simulink model "Flight_Simulation"  (R2021b)
settings: Solver=ode4  StartTime=0.0  StopTime=20  FixedStep=Settings.Simulation.step_size  RelTol=1e-3  EnableMultiTasking=on
undefined symbols (not defined in the file or in its folder): AeroCoeff, Aircraft, ControlGains, dLEF, Environment, F, Light, MIL, Settings, Trim, trim_control, trim_state, trim_thrust
libraries: simulink x19, simulink_extras x14, slpidlib x2, aerolibfltsims x2, aerolibwind2 x1, vrlib x1
(part 4 of 5)

== system Flight_Simulation/Non-linear_Plant/6DOF_Equations/Position_Differential_Equations/Calculate_north_position_dot ==
  U : Inport
  V : Inport  Port=2
  W : Inport  Port=3
  phi : Inport  Port=4
  theta : Inport  Port=5
  psi : Inport  Port=6
  Product3 : Product  Inputs=3
  Product4 : Product  Inputs=3
  Product{5..6,8..9} (4 alike) : Product
  Product7 : Product  Inputs=3
  Sum : Sum  Inputs=+-
  Sum1 : Sum
  Sum2 : Sum  Inputs=+++
  Trigonometric Function4 : Trigonometry  Operator=cos
  Trigonometric Function5 : Trigonometry  Operator=cos
  Trigonometric Function6 : Trigonometry
  Trigonometric Function7 : Trigonometry
  Trigonometric Function8 : Trigonometry  Operator=cos
  Trigonometric Function9 : Trigonometry
  north_pos_dot : Outport
  wires:
  phi/1 -> Trigonometric Function6/1, Trigonometric Function5/1
  Trigonometric Function7/1 -> Product7/2, Product4/3
  Product5/1 -> Sum/2
  V/1 -> Product6/1
  U/1 -> Product3/1
  W/1 -> Product9/1
  Trigonometric Function6/1 -> Product8/1, Product4/1
  psi/1 -> Trigonometric Function9/1, Trigonometric Function8/1
  Product3/1 -> Sum2/1
  Sum/1 -> Product6/2
  Trigonometric Function9/1 -> Product8/2, Product5/2
  Trigonometric Function8/1 -> Product4/2, Product3/3, Product7/3
  Trigonometric Function5/1 -> Product7/1, Product5/1
  Product7/1 -> Sum1/1
  Trigonometric Function4/1 -> Product3/2
  theta/1 -> Trigonometric Function7/1, Trigonometric Function4/1
  Sum1/1 -> Product9/2
  Product4/1 -> Sum/1
  Product9/1 -> Sum2/3
  Sum2/1 -> north_pos_dot/1  "north_pos_dot_m/s"
  Product6/1 -> Sum2/2
  Product8/1 -> Sum1/2

== system Flight_Simulation/Non-linear_Plant/6DOF_Equations/Position_Differential_Equations/Position_dot_WGS84 ==
  U_earth : Inport
  V_earth : Inport  Port=2
  alt_dot : Inport  Port=3
  Pos_WGS84 : Inport  Port=4
  Earth_Model_BUS : Inport  Port=5
  Bus Creator : BusCreator  Inputs=3
  Bus Selector : BusSelector  OutputSignals=R_Curvature_Meridian_m,R_Curvature_Prime_Vertical_m
  Bus Selector1 : BusSelector  OutputSignals=mue_pos_WGS84_rad,h_pos_WGS84_m
  Gain : Gain
  Product : Product
  Product1 : Product  Inputs=*/
  Product2 : Product  Inputs=*/
  Sum : Sum  Inputs=|++
  Sum1 : Sum
  Trigonometric Function : Trigonometry  Operator=cos
  Pos_WGS84_dot_BUS : Outport
  wires:
  Trigonometric Function/1 -> Product/1
  Sum/1 -> Product/2
  Bus Selector1/2 -> Sum1/1, Sum/1  "<h_pos_WGS84_m>"
  Bus Selector1/1 -> Trigonometric Function/1  "<mue_pos_WGS84_rad>"
  Product/1 -> Product1/2
  Earth_Model_BUS/1 -> Bus Selector/1
  Bus Selector/1 -> Sum1/2  "<R_Curvature_Meridian_m>"
  Bus Selector/2 -> Sum/2  "<R_Curvature_Prime_Vertical_m>"
  Sum1/1 -> Product2/2
  Product1/1 -> Bus Creator/1  "Pos_lambda_dot_WGS84_rad/s"
  Product2/1 -> Bus Creator/2  "Pos_mue_dot_WGS84_rad/s"
  Gain/1 -> Bus Creator/3  "Pos_h_dot_WGS84_m/s"
  Bus Creator/1 -> Pos_WGS84_dot_BUS/1  "Pos_WGS84_dot_BUS"
  V_earth/1 -> Product1/1
  U_earth/1 -> Product2/1
  alt_dot/1 -> Gain/1
  Pos_WGS84/1 -> Bus Selector1/1

== system Flight_Simulation/Non-linear_Plant/6DOF_Equations/Rotation_Differential_Equation/Inertia_Denominator_Calculation ==
  Aircraft_Constants_BUS : Inport
  Add : Sum  Inputs=+-
  Bus Selector : BusSelector  OutputSignals=Mass_Properties_BUS
  Bus Selector1 : BusSelector  OutputSignals=J_xx_kg*m^2,J_zz_kg*m^2,J_xz_kg*m^2
  Product : Product
  Product1 : Product
  Inertia_Denominator : Outport
  wires:
  Aircraft_Constants_BUS/1 -> Bus Selector/1
  Bus Selector/1 -> Bus Selector1/1  "<Mass_Properties_BUS>"
  Bus Selector1/1 -> Product/1  "<J_xx_kg*m^2>"
  Bus Selector1/2 -> Product/2  "<J_zz_kg*m^2>"
  Product/1 -> Add/1
  Bus Selector1/3 -> Product1/2, Product1/1  "<J_xz_kg*m^2>"
  Product1/1 -> Add/2
  Add/1 -> Inertia_Denominator/1

== system Flight_Simulation/Non-linear_Plant/6DOF_Equations/Rotation_Differential_Equation/p_dot_Calculation ==
  Moments_total_BUS : Inport
  Aircraft_Constants_BUS : Inport  Port=2
  States_BUS : Inport  Port=3
  Inertia_Denominator : Inport  Port=4
  Add : Sum  Inputs=++-++
  Add1 : Sum  Inputs=-+
  Add2 : Sum
  Add3 : Sum  Inputs=+-+
  Bus Selector : BusSelector  OutputSignals=Rates_p_q_r
  Bus Selector1 : BusSelector  OutputSignals=p_rad/s,q_rad/s,r_rad/s
  Bus Selector2 : BusSelector  OutputSignals=Engine_Const_BUS,Mass_Properties_BUS
  Bus Selector3 : BusSelector  OutputSignals=J_xx_kg*m^2,J_yy_kg*m^2,J_zz_kg*m^2,J_xz_kg*m^2
  Bus Selector4 : BusSelector  OutputSignals=L_total,N_total
  Bus Selector5 : BusSelector  OutputSignals=Engine_Ang_Mom_kg*m^2/s
  Divide : Product  Inputs=*/
  Product{,1..3} (4 alike) : Product
  Product4 : Product  Inputs=3
  Product5 : Product  Inputs=4
  Product6 : Product  Inputs=3
  p_dot : Outport
  wires:
  States_BUS/1 -> Bus Selector/1
  Bus Selector/1 -> Bus Selector1/1  "<Rates_p_q_r>"
  Aircraft_Constants_BUS/1 -> Bus Selector2/1
  Bus Selector2/2 -> Bus Selector3/1  "<Mass_Properties_BUS>"
  Moments_total_BUS/1 -> Bus Selector4/1
  Bus Selector3/4 -> Product6/3, Product5/2, Product3/1, Product3/2, Product1/1  "<J_xz_kg*m^2>"
  Bus Selector3/3 -> Add3/3, Product2/2, Add1/2, Product/1  "<J_zz_kg*m^2>"
  Bus Selector4/1 -> Product/2  "<L_total>"
  Bus Selector4/2 -> Product1/2  "<N_total>"
  Product/1 -> Add/4  "Jzz_L"
  Product1/1 -> Add/5  "Jxz_N"
  Add/1 -> Divide/1
  Bus Selector3/2 -> Add3/2, Add1/1  "<J_yy_kg*m^2>"
  Add1/1 -> Product2/1
  Product2/1 -> Add2/2
  Product3/1 -> Add2/1
  Add2/1 -> Product4/3
  Bus Selector1/2 -> Product6/2, Product5/4, Product4/1  "<q_rad/s>"
  Bus Selector1/3 -> Product4/2  "<r_rad/s>"
  Product4/1 -> Add/3  "QR_term"
  Bus Selector3/1 -> Add3/1  "<J_xx_kg*m^2>"
  Add3/1 -> Product5/1
  Bus Selector1/1 -> Product5/3  "<p_rad/s>"
  Product5/1 -> Add/2  "PQ_term"
  Product6/1 -> Add/1
  Bus Selector2/1 -> Bus Selector5/1  "<Engine_Const_BUS>"
  Bus Selector5/1 -> Product6/1  "<Engine_Ang_Mom_kg*m^2/s>"
  Inertia_Denominator/1 -> Divide/2
  Divide/1 -> p_dot/1  "p_dot_rad/s^2"

== system Flight_Simulation/Non-linear_Plant/6DOF_Equations/Rotation_Differential_Equation/q_dot_Calculation ==
  note: * Momentum_engine_angular
  States_BUS : Inport
  Aircraft_Constants_BUS : Inport  Port=2
  Moments_total_BUS : Inport  Port=3
  Engine_BUS : Inport  Port=4
  Add : Sum  Inputs=-+-+
  Add1 : Sum  Inputs=-+
  Add2 : Sum  Inputs=+-
  Bus Selector : BusSelector  OutputSignals=Rates_p_q_r
  Bus Selector1 : BusSelector  OutputSignals=p_rad/s,r_rad/s
  Bus Selector2 : BusSelector  OutputSignals=Engine_Const_BUS,Mass_Properties_BUS
  Bus Selector3 : BusSelector  OutputSignals=J_xx_kg*m^2,J_zz_kg*m^2,J_xz_kg*m^2,J_yy_kg*m^2
  Bus Selector4 : BusSelector  OutputSignals=M_total
  Bus Selector5 : BusSelector  OutputSignals=Engine_Ang_Mom_kg*m^2/s
  Bus Selector6 : BusSelector  OutputSignals=M_engine_Nm
  Divide : Product  Inputs=*/
  Product : Product  Inputs=3
  Product{1..4} (4 alike) : Product
  Sum : Sum  Inputs=|++
  q_dot : Outport
  wires:
  Divide/1 -> q_dot/1  "q_dot_rad/s^2"
  Bus Selector2/1 -> Bus Selector5/1  "<Engine_Const_BUS>"
  Add/1 -> Divide/1
  Moments_total_BUS/1 -> Bus Selector4/1
  Bus Selector2/2 -> Bus Selector3/1  "<Mass_Properties_BUS>"
  Aircraft_Constants_BUS/1 -> Bus Selector2/1
  Bus Selector/1 -> Bus Selector1/1  "<Rates_p_q_r>"
  States_BUS/1 -> Bus Selector/1
  Bus Selector4/1 -> Sum/1  "<M_total>"
  Bus Selector3/1 -> Add1/1  "<J_xx_kg*m^2>"
  Bus Selector3/2 -> Add1/2  "<J_zz_kg*m^2>"
  Add1/1 -> Product/3
  Bus Selector1/1 -> Product2/1, Product2/2, Product/1  "<p_rad/s>"
  Bus Selector1/2 -> Product4/2, Product3/1, Product3/2, Product/2  "<r_rad/s>"
  Product/1 -> Add/2  "PR_term"
  Bus Selector3/3 -> Product1/2  "<J_xz_kg*m^2>"
  Product2/1 -> Add2/1
  Product3/1 -> Add2/2
  Add2/1 -> Product1/1
  Product1/1 -> Add/3  "jxz_term"
  Bus Selector5/1 -> Product4/1  "<Engine_Ang_Mom_kg*m^2/s>"
  Product4/1 -> Add/1
  Bus Selector3/4 -> Divide/2  "<J_yy_kg*m^2>"
  Sum/1 -> Add/4  "M_total+M_engine"
  Engine_BUS/1 -> Bus Selector6/1
  Bus Selector6/1 -> Sum/2  "<M_engine_Nm>"

== system Flight_Simulation/Non-linear_Plant/6DOF_Equations/Rotation_Differential_Equation/r_dot_Calculation ==
  Inertia_Denominator : Inport
  States_BUS : Inport  Port=2
  Aircraft_Constants_BUS : Inport  Port=3
  Moments_total_BUS : Inport  Port=4
  Add : Sum  Inputs=+-+++
  Add1 : Sum  Inputs=+-
  Add2 : Sum
  Add3 : Sum  Inputs=+-+
  Bus Selector : BusSelector  OutputSignals=Rates_p_q_r
  Bus Selector1 : BusSelector  OutputSignals=p_rad/s,q_rad/s,r_rad/s
  Bus Selector2 : BusSelector  OutputSignals=Engine_Const_BUS,Mass_Properties_BUS
  Bus Selector3 : BusSelector  OutputSignals=J_xx_kg*m^2,J_yy_kg*m^2,J_zz_kg*m^2,J_xz_kg*m^2
  Bus Selector4 : BusSelector  OutputSignals=L_total,N_total
  Bus Selector5 : BusSelector  OutputSignals=Engine_Ang_Mom_kg*m^2/s
  Divide : Product  Inputs=*/
  Product{,1..3} (4 alike) : Product
  Product4 : Product  Inputs=3
  Product5 : Product  Inputs=4
  Product6 : Product  Inputs=3
  r_dot : Outport
  wires:
  Divide/1 -> r_dot/1  "r_dot_rad/s^2"
  Inertia_Denominator/1 -> Divide/2
  Bus Selector5/1 -> Product6/1  "<Engine_Ang_Mom_kg*m^2/s>"
  Bus Selector2/1 -> Bus Selector5/1  "<Engine_Const_BUS>"
  Product6/1 -> Add/1
  Product5/1 -> Add/2
  Add3/1 -> Product5/1
  Product4/1 -> Add/3  "PQ_Term"
  Add2/1 -> Product4/3
  Product3/1 -> Add2/1
  Product2/1 -> Add2/2
  Add1/1 -> Product2/1
  Add/1 -> Divide/1
  Product1/1 -> Add/5  "Jx_N"
  Product/1 -> Add/4  "Jxz_L"
  Moments_total_BUS/1 -> Bus Selector4/1
  Bus Selector2/2 -> Bus Selector3/1  "<Mass_Properties_BUS>"
  Aircraft_Constants_BUS/1 -> Bus Selector2/1
  Bus Selector/1 -> Bus Selector1/1  "<Rates_p_q_r>"
  States_BUS/1 -> Bus Selector/1
  Bus Selector4/2 -> Product1/2  "<N_total>"
  Bus Selector3/1 -> Product6/3, Add3/1, Add1/1, Product2/2, Product1/1  "<J_xx_kg*m^2>"
  Bus Selector3/4 -> Product5/4, Product3/1, Product3/2, Product/1  "<J_xz_kg*m^2>"
  Bus Selector4/1 -> Product/2  "<L_total>"
  Bus Selector3/2 -> Add3/2, Add1/2  "<J_yy_kg*m^2>"
  Bus Selector1/1 -> Product4/1  "<p_rad/s>"
  Bus Selector1/2 -> Product6/2, Product5/2, Product4/2  "<q_rad/s>"
  Bus Selector3/3 -> Add3/3  "<J_zz_kg*m^2>"
  Bus Selector1/3 -> Product5/3  "<r_rad/s>"

== system Flight_Simulation/Non-linear_Plant/6DOF_Equations/Translation_UVW_Differential_Equations/U_dot ==
  States_BUS : Inport
  Forces_total_BUS : Inport  Port=2
  Aircraft_Constants_BUS : Inport  Port=3
  Gravity_BUS : Inport  Port=4
  Engine_BUS : Inport  Port=5
  Bus Selector : BusSelector  OutputSignals=Angles_phi_theta_psi
  Bus Selector1 : BusSelector  OutputSignals=theta_rad
  Bus Selector10 : BusSelector  OutputSignals=X_total
  Bus Selector11 : BusSelector  OutputSignals=Thrust_act_N
  Bus Selector2 : BusSelector  OutputSignals=g_m/s^2
  Bus Selector3 : BusSelector  OutputSignals=Rates_p_q_r
  Bus Selector4 : BusSelector  OutputSignals=q_rad/s,r_rad/s
  Bus Selector5 : BusSelector  OutputSignals=V_m/s,W_m/s
  Bus Selector6 : BusSelector  OutputSignals=Vel_U_V_W_body
  Bus Selector9 : BusSelector  OutputSignals=Mass_Properties_BUS.Mass_kg
  Divide : Product  Inputs=/*
  Divide1 : Product  Inputs=*/
  Product : Product
  Product1 : Product
  Product2 : Product
  Sum : Sum  Inputs=--+++
  Trigonometric Function : Trigonometry
  U_dot : Outport
  wires:
  Sum/1 -> U_dot/1  "U_dot"
  States_BUS/1 -> Bus Selector3/1, Bus Selector6/1, Bus Selector/1
  Bus Selector/1 -> Bus Selector1/1  "<Angles_phi_theta_psi>"
  Bus Selector1/1 -> Trigonometric Function/1  "<theta_rad>"
  Gravity_BUS/1 -> Bus Selector2/1
  Bus Selector2/1 -> Product/1  "<g_m/s^2>"
  Trigonometric Function/1 -> Product/2
  Product/1 -> Sum/1
  Bus Selector3/1 -> Bus Selector4/1  "<Rates_p_q_r>"
  Bus Selector4/1 -> Product2/1  "<q_rad/s>"
  Bus Selector4/2 -> Product1/1  "<r_rad/s>"
  Bus Selector5/1 -> Product1/2  "<V_m/s>"
  Product1/1 -> Sum/3
  Bus Selector5/2 -> Product2/2  "<W_m/s>"
  Product2/1 -> Sum/2
  Aircraft_Constants_BUS/1 -> Bus Selector9/1
  Bus Selector9/1 -> Divide1/2, Divide/1  "<Mass_kg>"
  Forces_total_BUS/1 -> Bus Selector10/1
  Engine_BUS/1 -> Bus Selector11/1
  Bus Selector11/1 -> Divide1/1  "<Thrust_act_N>"
  Bus Selector10/1 -> Divide/2  "<X_total>"
  Divide/1 -> Sum/5
  Divide1/1 -> Sum/4
  Bus Selector6/1 -> Bus Selector5/1  "<Vel_U_V_W_body>"

== system Flight_Simulation/Non-linear_Plant/6DOF_Equations/Translation_UVW_Differential_Equations/V_dot ==
  States_BUS : Inport
  Forces_total_BUS : Inport  Port=2
  Aircraft_Constants_BUS1 : Inport  Port=3
  Gravity_BUS : Inport  Port=4
  Bus Selector : BusSelector  OutputSignals=Angles_phi_theta_psi
  Bus Selector1 : BusSelector  OutputSignals=phi_rad,theta_rad
  Bus Selector11 : BusSelector  OutputSignals=Y_total
  Bus Selector12 : BusSelector  OutputSignals=Mass_Properties_BUS.Mass_kg
  Bus Selector2 : BusSelector  OutputSignals=g_m/s^2
  Bus Selector3 : BusSelector  OutputSignals=Rates_p_q_r
  Bus Selector4 : BusSelector  OutputSignals=p_rad/s,r_rad/s
  Bus Selector5 : BusSelector  OutputSignals=U_m/s,W_m/s
  Bus Selector6 : BusSelector  OutputSignals=Vel_U_V_W_body
  Divide1 : Product  Inputs=/*
  Product : Product  Inputs=3
  Product1 : Product
  Product2 : Product
  Sum : Sum  Inputs=++-+
  Trigonometric Function : Trigonometry
  Trigonometric Function1 : Trigonometry  Operator=cos
  V_dot : Outport
  wires:
  Sum/1 -> V_dot/1  "V_dot"
  States_BUS/1 -> Bus Selector6/1, Bus Selector3/1, Bus Selector/1
  Bus Selector/1 -> Bus Selector1/1  "<Angles_phi_theta_psi>"
  Bus Selector1/2 -> Trigonometric Function1/1  "<theta_rad>"
  Gravity_BUS/1 -> Bus Selector2/1
  Bus Selector2/1 -> Product/1  "<g_m/s^2>"
  Trigonometric Function/1 -> Product/2
  Product/1 -> Sum/1  "g_ct_sphi"
  Bus Selector3/1 -> Bus Selector4/1  "<Rates_p_q_r>"
  Bus Selector4/1 -> Product2/1  "<p_rad/s>"
  Bus Selector4/2 -> Product1/1  "<r_rad/s>"
  Bus Selector5/1 -> Product1/2  "<U_m/s>"
  Product1/1 -> Sum/3  "RU"
  Bus Selector5/2 -> Product2/2  "<W_m/s>"
  Product2/1 -> Sum/2  "PW"
  Trigonometric Function1/1 -> Product/3
  Bus Selector1/1 -> Trigonometric Function/1  "<phi_rad>"
  Divide1/1 -> Sum/4  "qbar_S_Cy_m"
  Forces_total_BUS/1 -> Bus Selector11/1
  Bus Selector12/1 -> Divide1/1  "<Mass_kg>"
  Bus Selector11/1 -> Divide1/2  "<Y_total>"
  Aircraft_Constants_BUS1/1 -> Bus Selector12/1
  Bus Selector6/1 -> Bus Selector5/1  "<Vel_U_V_W_body>"

== system Flight_Simulation/Non-linear_Plant/6DOF_Equations/Translation_UVW_Differential_Equations/W_dot ==
  States_BUS : Inport
  Force_Coeff_BUS : Inport  Port=2
  Aircraft_Constants_BUS : Inport  Port=3
  Gravity_BUS : Inport  Port=4
  Bus Selector : BusSelector  OutputSignals=Angles_phi_theta_psi
  Bus Selector1 : BusSelector  OutputSignals=phi_rad,theta_rad
  Bus Selector10 : BusSelector  OutputSignals=Z_total
  Bus Selector2 : BusSelector  OutputSignals=g_m/s^2
  Bus Selector3 : BusSelector  OutputSignals=Rates_p_q_r
  Bus Selector4 : BusSelector  OutputSignals=q_rad/s,p_rad/s
  Bus Selector5 : BusSelector  OutputSignals=V_m/s,U_m/s
  Bus Selector6 : BusSelector  OutputSignals=Vel_U_V_W_body
  Bus Selector9 : BusSelector  OutputSignals=Mass_Properties_BUS.Mass_kg
  Divide : Product  Inputs=*/
  Product : Product  Inputs=3
  Product1 : Product
  Product2 : Product
  Sum : Sum  Inputs=++-+
  Trigonometric Function : Trigonometry  Operator=cos
  Trigonometric Function1 : Trigonometry  Operator=cos
  W_dot : Outport
  wires:
  Aircraft_Constants_BUS/1 -> Bus Selector9/1
  Product2/1 -> Sum/2  "UQ"
  Bus Selector5/2 -> Product2/2  "<U_m/s>"
  Product1/1 -> Sum/3  "VP"
  Bus Selector5/1 -> Product1/2  "<V_m/s>"
  Bus Selector4/2 -> Product1/1  "<p_rad/s>"
  Bus Selector4/1 -> Product2/1  "<q_rad/s>"
  Bus Selector3/1 -> Bus Selector4/1  "<Rates_p_q_r>"
  Product/1 -> Sum/1  "g_ctheta_cphi"
  Trigonometric Function/1 -> Product/3
  Bus Selector2/1 -> Product/1  "<g_m/s^2>"
  Gravity_BUS/1 -> Bus Selector2/1
  Bus Selector1/2 -> Trigonometric Function/1  "<theta_rad>"
  Bus Selector/1 -> Bus Selector1/1  "<Angles_phi_theta_psi>"
  States_BUS/1 -> Bus Selector/1, Bus Selector6/1, Bus Selector3/1
  Sum/1 -> W_dot/1  "W_dot"
  Divide/1 -> Sum/4  "Z_total/m"
  Bus Selector1/1 -> Trigonometric Function1/1  "<phi_rad>"
  Trigonometric Function1/1 -> Product/2
  Bus Selector9/1 -> Divide/2  "<Mass_kg>"
  Bus Selector10/1 -> Divide/1  "<Z_total>"
  Force_Coeff_BUS/1 -> Bus Selector10/1
  Bus Selector6/1 -> Bus Selector5/1  "<Vel_U_V_W_body>"

== system Flight_Simulation/Non-linear_Plant/Actuator_Models/Leading Edge Flap/LEF Actuator ==
  In1 : Inport
  Command Saturation : Saturate  UpperLimit=25  LowerLimit=0
  Gain : Gain  Gain=1/0.136  SaturateOnIntegerOverflow=on  OutDataTypeStr=Inherit: Same as input  ParamDataTypeStr=Inherit: Same as input
  "LF_pos_int " : Integrator  InitialConditionSource=external  InitialCondition=dLEF  UpperSaturationLimit=21.5  LowerSaturationLimit=-21.5
  Rate Saturation : Saturate  UpperLimit=25  LowerLimit=-25
  Sum : Sum  Inputs=|+-  InputSameDT=on  SaturateOnIntegerOverflow=on  OutDataTypeStr=Inherit: Same as first input
  Out1 : Outport
  wires:
  "LF_pos_int "/1 -> Sum/2, Out1/1
  Rate Saturation/1 -> "LF_pos_int "/1
  Gain/1 -> Rate Saturation/1
  Sum/1 -> Gain/1
  Command Saturation/1 -> Sum/1
  In1/1 -> Command Saturation/1, "LF_pos_int "/2

== system Flight_Simulation/Non-linear_Plant/Aerodynamic_Modul/Aero_Coefficients/Controls unit preparation ==
  Controls_BUS : Inport
  Bus Creator1 : BusCreator  Inputs=4
  Bus Selector1 : BusSelector  OutputSignals=Elevator_act_deg,Aileron_act_deg,Rudder_act_deg,Speedbrakes_cmd_%
  Constant : Constant  Value=AeroCoeff.SwitchDegree.control_angles
  Degrees to Radians : simulink_extras/Transformations/Degrees to Radians
  Demux : Demux  Outputs=3
  Mux : Mux  Inputs=3
  Switch : Switch  Criteria=u2 > Threshold
  prep_Controls_BUS : Outport
  wires:
  Controls_BUS/1 -> Bus Selector1/1
  Bus Selector1/3 -> Mux/3  "<Rudder_act_deg>"
  Bus Creator1/1 -> prep_Controls_BUS/1  "Controls_BUS"
  Bus Selector1/2 -> Mux/2  "<Aileron_act_deg>"
  Bus Selector1/1 -> Mux/1  "<Elevator_act_deg>"
  Demux/1 -> Bus Creator1/1  "Elevator_act"
  Demux/2 -> Bus Creator1/2  "Aileron_act"
  Demux/3 -> Bus Creator1/3  "Rudder_act"
  Bus Selector1/4 -> Bus Creator1/4  "<Speedbrakes_cmd_%>"
  Mux/1 -> Degrees to Radians/1, Switch/1
  Constant/1 -> Switch/2
  Switch/1 -> Demux/1
  Degrees to Radians/1 -> Switch/3

== system Flight_Simulation/Non-linear_Plant/Aerodynamic_Modul/Aero_Coefficients/Force_Coefficients ==
  Atmosphere_BUS : Inport
  States_BUS : Inport  Port=2
  alpha_beta : Inport  Port=3
  Aircraft_Constant_BUS : Inport  Port=4
  prep_Controls_BUS : Inport  Port=5
  Engine_BUS : Inport  Port=6
  Bus Creator1 : BusCreator  Inputs=3
  C_x_total : Subsystem
  C_y_total : Subsystem
  C_z_total : Subsystem
  Force_Coeff_BUS : Outport
  wires:
  C_x_total/1(C_x_total) -> Bus Creator1/1  "C_x_total"
  States_BUS/1 -> C_x_total/2(States_BUS), C_z_total/1(States_BUS), C_y_total/1(States_BUS)
  C_y_total/1(C_y_total) -> Bus Creator1/2  "C_y_total"
  Bus Creator1/1 -> Force_Coeff_BUS/1  "Force_Coeff_BUS"
  C_z_total/1(C_z_total) -> Bus Creator1/3  "C_z_total"
  Aircraft_Constant_BUS/1 -> C_x_total/4(Aircraft_Constant_BUS), C_z_total/3(Aircraft_Constant_BUS), C_y_total/3(Aircraft_Constant_BUS)
  Engine_BUS/1 -> C_z_total/5(Engine_BUS), C_x_total/6(Engine_BUS)
  prep_Controls_BUS/1 -> C_x_total/5(prep_Controls_BUS), C_z_total/4(prep_Controls_BUS), C_y_total/4(prep_Controls_BUS)
  alpha_beta/1 -> C_x_total/3(alpha_beta), C_z_total/2(alpha_beta), C_y_total/2(alpha_beta)
  Atmosphere_BUS/1 -> C_x_total/1(Atmosphere_BUS)

== system Flight_Simulation/Non-linear_Plant/Aerodynamic_Modul/Aero_Coefficients/Moment_Coefficients ==
  Force_Coefficients : Inport
  States_BUS : Inport  Port=2
  alpha_beta : Inport  Port=3
  Aircraft_Constant_BUS : Inport  Port=4
  prep_Controls_BUS : Inport  Port=5
  Engine_BUS : Inport  Port=6
  Bus Creator2 : BusCreator  Inputs=3
  C_l_total : Subsystem
  C_m_total : Subsystem
  C_n_total : Subsystem
  Moment_Coeff_BUS : Outport
  wires:
  Force_Coefficients/1 -> C_n_total/5(Force_Coefficients), C_m_total/6(Force_Coefficients)
  C_n_total/1(C_n_total) -> Bus Creator2/3
  C_l_total/1(C_l_total) -> Bus Creator2/1
  alpha_beta/1 -> C_n_total/2(alpha_beta), C_m_total/2(alpha_beta), C_l_total/2(alpha_beta)
  prep_Controls_BUS/1 -> C_n_total/4(prep_Controls_BUS), C_m_total/4(prep_Controls_BUS), C_l_total/4(prep_Controls_BUS)
  C_m_total/1(C_m_total) -> Bus Creator2/2
  Aircraft_Constant_BUS/1 -> C_n_total/3(Aircraft_Constant_BUS), C_m_total/3(Aircraft_Constant_BUS), C_l_total/3(Aircraft_Constant_BUS)
  States_BUS/1 -> C_l_total/1(States_BUS), C_n_total/1(States_BUS), C_m_total/1(States_BUS)
  Engine_BUS/1 -> C_m_total/5(Engine_BUS)
  Bus Creator2/1 -> Moment_Coeff_BUS/1  "Moment_Coeff_BUS"

== system Flight_Simulation/Non-linear_Plant/Aerodynamic_Modul/Aero_Coefficients/alpha beta unit preparation ==
  States_BUS : Inport
  Bus Creator : BusCreator  Inputs=2
  Bus Selector : BusSelector  OutputSignals=Vel_aero_V_alpha_beta.alpha_rad,Vel_aero_V_alpha_beta.beta_rad
  Constant : Constant  Value=AeroCoeff.SwitchDegree.alpha_beta
  Demux : Demux  Outputs=2
  Mux : Mux  Inputs=2
  Radians to Degrees : simulink_extras/Transformations/Radians to Degrees
  Switch : Switch  Criteria=u2 > Threshold
  alpha_beta : Outport
  wires:
  Bus Selector/1 -> Mux/1  "<alpha_rad>"
  Bus Selector/2 -> Mux/2  "<beta_rad>"
  States_BUS/1 -> Bus Selector/1
  Demux/1 -> Bus Creator/1  "alpha"
  Demux/2 -> Bus Creator/2  "beta"
  Bus Creator/1 -> alpha_beta/1
  Mux/1 -> Switch/3, Radians to Degrees/1
  Constant/1 -> Switch/2
  Switch/1 -> Demux/1
  Radians to Degrees/1 -> Switch/1

== system Flight_Simulation/Non-linear_Plant/Aerodynamic_Modul/Total Aero Moments/L_total_Calculation ==
  Atmosphere_BUS : Inport
  Aircraft_Constants_BUS : Inport  Port=2
  Moment_Coeff_BUS : Inport  Port=3
  Bus Selector : BusSelector  OutputSignals=C_l_total
  Bus Selector1 : BusSelector  OutputSignals=q_bar_Pa
  Bus Selector3 : BusSelector  OutputSignals=Wing_Dimension_BUS.WingSpan_m,Wing_Dimension_BUS.WingArea_m^2
  Product : Product  Inputs=4
  L_total : Outport
  wires:
  Atmosphere_BUS/1 -> Bus Selector1/1
  Bus Selector/1 -> Product/4  "<C_l_total>"
  Moment_Coeff_BUS/1 -> Bus Selector/1
  Bus Selector1/1 -> Product/1  "<q_bar_Pa>"
  Bus Selector3/1 -> Product/2  "<WingSpan_m>"
  Product/1 -> L_total/1  "L_total"
  Aircraft_Constants_BUS/1 -> Bus Selector3/1
  Bus Selector3/2 -> Product/3  "<WingArea_m^2>"

== system Flight_Simulation/Non-linear_Plant/Aerodynamic_Modul/Total Aero Moments/M_total_Calculation ==
  Atmosphere_BUS : Inport
  Aircraft_Constants_BUS : Inport  Port=2
  Moment_Coeff_BUS : Inport  Port=3
  Bus Selector : BusSelector  OutputSignals=C_m_total
  Bus Selector1 : BusSelector  OutputSignals=q_bar_Pa
  Bus Selector3 : BusSelector  OutputSignals=Wing_Dimension_BUS.MAC_m,Wing_Dimension_BUS.WingArea_m^2
  Product : Product  Inputs=4
  M_total : Outport
  wires:
  Bus Selector3/2 -> Product/3  "<WingArea_m^2>"
  Aircraft_Constants_BUS/1 -> Bus Selector3/1
  Bus Selector3/1 -> Product/2  "<MAC_m>"
  Bus Selector1/1 -> Product/1  "<q_bar_Pa>"
  Moment_Coeff_BUS/1 -> Bus Selector/1
  Bus Selector/1 -> Product/4  "<C_m_total>"
  Atmosphere_BUS/1 -> Bus Selector1/1
  Product/1 -> M_total/1  "M_total"

== system Flight_Simulation/Non-linear_Plant/Aerodynamic_Modul/Total Aero Moments/N_total_Calculation ==
  Atmosphere_BUS : Inport
  Aircraft_Constants_BUS : Inport  Port=2
  Moment_Coeff_BUS : Inport  Port=3
  Bus Selector : BusSelector  OutputSignals=C_n_total
  Bus Selector1 : BusSelector  OutputSignals=q_bar_Pa
  Bus Selector3 : BusSelector  OutputSignals=Wing_Dimension_BUS.WingSpan_m,Wing_Dimension_BUS.WingArea_m^2
  Product : Product  Inputs=4
  N_total : Outport
  wires:
  Atmosphere_BUS/1 -> Bus Selector1/1
  Moment_Coeff_BUS/1 -> Bus Selector/1
  Bus Selector1/1 -> Product/1  "<q_bar_Pa>"
  Bus Selector3/1 -> Product/2  "<WingSpan_m>"
  Product/1 -> N_total/1  "N_total"
  Aircraft_Constants_BUS/1 -> Bus Selector3/1
  Bus Selector/1 -> Product/4  "<C_n_total>"
  Bus Selector3/2 -> Product/3  "<WingArea_m^2>"

== system Flight_Simulation/Environment_Subsystems/Wind_Model/Gust_model_(1-cos)/reset flags after gust/Triggered Subsystem ==
  Trigger : TriggerPort  VariantControl=Variant  ShowOutputPort=on
  u_flg : Outport
  wires:
  Trigger/1 -> u_flg/1

== system Flight_Simulation/Environment_Subsystems/Wind_Model/Gust_model_(1-cos)/reset flags after gust/Triggered Subsystem1 ==
  Trigger : TriggerPort  VariantControl=Variant  ShowOutputPort=on
  v_flg : Outport
  wires:
  Trigger/1 -> v_flg/1

== system Flight_Simulation/Environment_Subsystems/Wind_Model/Gust_model_(1-cos)/reset flags after gust/Triggered Subsystem2 ==
  Trigger : TriggerPort  VariantControl=Variant  ShowOutputPort=on
  w_flg : Outport
  wires:
  Trigger/1 -> w_flg/1

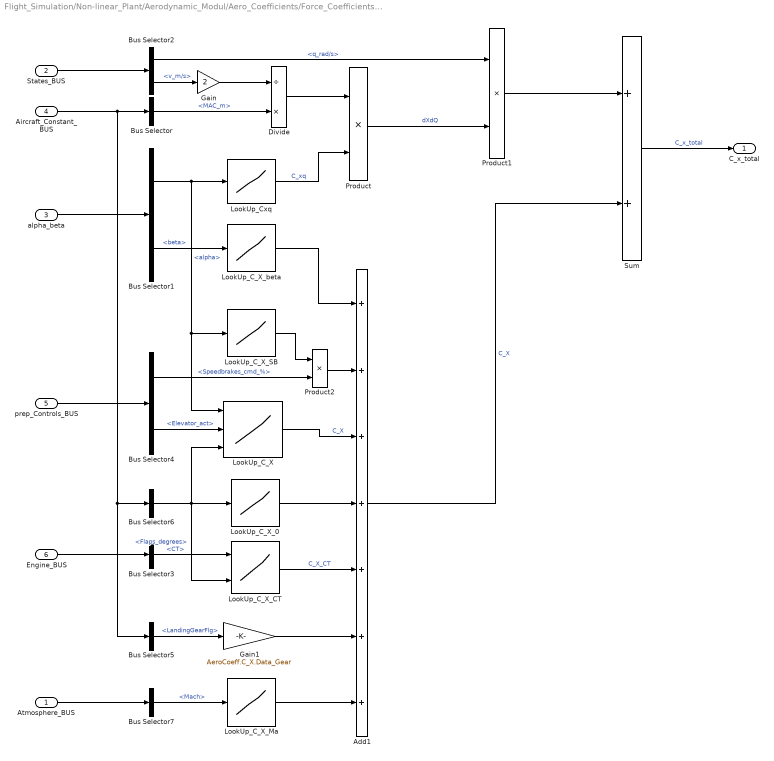
== system Flight_Simulation/Non-linear_Plant/Aerodynamic_Modul/Aero_Coefficients/Force_Coefficients/C_x_total ==
  Atmosphere_BUS : Inport
  States_BUS : Inport  Port=2
  alpha_beta : Inport  Port=3
  Aircraft_Constant_BUS : Inport  Port=4
  prep_Controls_BUS : Inport  Port=5
  Engine_BUS : Inport  Port=6
  Add1 : Sum  Inputs=+++++++
  Bus Selector : BusSelector  OutputSignals=Wing_Dimension_BUS.MAC_m
  Bus Selector1 : BusSelector  OutputSignals=alpha,beta
  Bus Selector2 : BusSelector  OutputSignals=Rates_p_q_r.q_rad/s,Vel_aero_V_alpha_beta.v_m/s
  Bus Selector3 : BusSelector  OutputSignals=CT
  Bus Selector4 : BusSelector  OutputSignals=Speedbrakes_cmd_%,Elevator_act
  Bus Selector5 : BusSelector  OutputSignals=LandingGearFlg
  Bus Selector6 : BusSelector  OutputSignals=Flaps_degrees
  Bus Selector7 : BusSelector  OutputSignals=Mach
  Divide : Product  Inputs=/*
  Gain : Gain  Gain=2
  Gain1 : Gain  Gain=AeroCoeff.C_X.Data_Gear
  LookUp_C_X : Lookup_n-D  NumberOfTableDimensions=3  BreakpointsForDimension1=AeroCoeff.C_X.alpha  BreakpointsForDimension2=AeroCoeff.C_X.eta  BreakpointsForDimension3=AeroCoeff.C_X.Flaps  Table=AeroCoeff.C_X.Data_alphaeta  InternalRulePriority=Speed  RndMeth=Simplest  InputSameDT=on
      settings: InputPortMap=u0,u1,u2
  LookUp_C_X_0 : Lookup_n-D  NumberOfTableDimensions=1  BreakpointsForDimension1=AeroCoeff.C_X.Flaps  Table=AeroCoeff.C_X.Data_0  InternalRulePriority=Speed  RndMeth=Simplest  InputSameDT=on
  LookUp_C_X_CT : Lookup_n-D  BreakpointsForDimension1=AeroCoeff.C_X.CT  BreakpointsForDimension2=AeroCoeff.C_X.Flaps  Table=AeroCoeff.C_X.Data_CT_Fl  InternalRulePriority=Speed  RndMeth=Simplest  InputSameDT=on
      settings: InputPortMap=u0,u1
  LookUp_C_X_Ma : Lookup_n-D  NumberOfTableDimensions=1  BreakpointsForDimension1=AeroCoeff.C_X.Mach  Table=AeroCoeff.C_X.Data_Mach  InternalRulePriority=Speed  RndMeth=Simplest  InputSameDT=on
  LookUp_C_X_SB : Lookup_n-D  NumberOfTableDimensions=1  BreakpointsForDimension1=AeroCoeff.C_X.alpha  Table=AeroCoeff.C_X.Data_sb_alpha  InternalRulePriority=Speed  RndMeth=Simplest  InputSameDT=on
  LookUp_C_X_beta : Lookup_n-D  NumberOfTableDimensions=1  BreakpointsForDimension1=AeroCoeff.C_X.beta  Table=AeroCoeff.C_X.Data_beta  InternalRulePriority=Speed  RndMeth=Simplest  InputSameDT=on
  LookUp_Cxq : Lookup_n-D  NumberOfTableDimensions=1  BreakpointsForDimension1=AeroCoeff.C_xq.alpha  Table=AeroCoeff.C_xq.Data  DiagnosticForOutOfRangeInput=Warning  InternalRulePriority=Speed  RndMeth=Simplest  InputSameDT=on
  Product : Product
  Product1 : Product
  Product2 : Product
  Sum : Sum
  C_x_total : Outport
  wires:
  States_BUS/1 -> Bus Selector2/1
  Aircraft_Constant_BUS/1 -> Bus Selector/1, Bus Selector5/1, Bus Selector6/1
  Bus Selector2/2 -> Gain/1  "<v_m/s>"
  Gain/1 -> Divide/1
  Bus Selector/1 -> Divide/2  "<MAC_m>"
  Divide/1 -> Product/1
  Product/1 -> Product1/2  "dXdQ"
  Add1/1 -> Sum/2  "C_X"
  Bus Selector2/1 -> Product1/1  "<q_rad/s>"
  Product1/1 -> Sum/1
  Sum/1 -> C_x_total/1  "C_x_total"
  LookUp_Cxq/1 -> Product/2  "C_xq"
  alpha_beta/1 -> Bus Selector1/1
  Bus Selector1/1 -> LookUp_Cxq/1, LookUp_C_X/1, LookUp_C_X_SB/1  "<alpha>"
  LookUp_C_X/1 -> Add1/3  "C_X"
  LookUp_C_X_CT/1 -> Add1/5  "C_X_CT"
  Engine_BUS/1 -> Bus Selector3/1
  Bus Selector4/2 -> LookUp_C_X/2  "<Elevator_act>"
  Bus Selector3/1 -> LookUp_C_X_CT/1  "<CT>"
  prep_Controls_BUS/1 -> Bus Selector4/1
  Gain1/1 -> Add1/6
  Bus Selector5/1 -> Gain1/1  "<LandingGearFlg>"
  Bus Selector1/2 -> LookUp_C_X_beta/1  "<beta>"
  LookUp_C_X_beta/1 -> Add1/1
  LookUp_C_X_0/1 -> Add1/4
  Bus Selector6/1 -> LookUp_C_X/3, LookUp_C_X_CT/2, LookUp_C_X_0/1  "<Flaps_degrees>"
  Atmosphere_BUS/1 -> Bus Selector7/1
  Bus Selector7/1 -> LookUp_C_X_Ma/1  "<Mach>"
  LookUp_C_X_Ma/1 -> Add1/7
  LookUp_C_X_SB/1 -> Product2/1
  Bus Selector4/1 -> Product2/2  "<Speedbrakes_cmd_%>"
  Product2/1 -> Add1/2

== system Flight_Simulation/Non-linear_Plant/Aerodynamic_Modul/Aero_Coefficients/Force_Coefficients/C_y_total ==
  States_BUS : Inport
  alpha_beta : Inport  Port=2
  Aircraft_Constant_BUS : Inport  Port=3
  prep_Controls_BUS : Inport  Port=4
  Add1 : Sum  Inputs=++++
  Bus Selector : BusSelector  OutputSignals=Wing_Dimension_BUS.WingSpan_m
  Bus Selector2 : BusSelector  OutputSignals=Rates_p_q_r.p_rad/s,Rates_p_q_r.r_rad/s,Vel_aero_V_alpha_beta.v_m/s
  Bus Selector3 : BusSelector  OutputSignals=alpha,beta
  Bus Selector4 : BusSelector  OutputSignals=Aileron_act,Rudder_act
  C_Y0 : Constant  Value=AeroCoeff.C_Y0
  Divide : Product  Inputs=/*
  Gain : Gain  Gain=2
  LookUp_CYp : Lookup_n-D  NumberOfTableDimensions=1  BreakpointsForDimension1=AeroCoeff.C_yp.alpha  Table=AeroCoeff.C_yp.Data  InternalRulePriority=Speed  RndMeth=Simplest  InputSameDT=on
  LookUp_CYr : Lookup_n-D  NumberOfTableDimensions=1  BreakpointsForDimension1=AeroCoeff.C_yr.alpha  Table=AeroCoeff.C_yr.Data  InternalRulePriority=Speed  RndMeth=Simplest  InputSameDT=on
  LookUp_C_Y_ail : Lookup_n-D  NumberOfTableDimensions=1  BreakpointsForDimension1=AeroCoeff.C_Y.ail  Table=AeroCoeff.C_Y.Data_ail  InternalRulePriority=Speed  RndMeth=Simplest  InputSameDT=on
  LookUp_C_Y_beta : Lookup_n-D  NumberOfTableDimensions=1  BreakpointsForDimension1=AeroCoeff.C_Y.beta  Table=AeroCoeff.C_Y.Data_beta  InternalRulePriority=Speed  RndMeth=Simplest  InputSameDT=on
  LookUp_C_Y_rud : Lookup_n-D  NumberOfTableDimensions=1  BreakpointsForDimension1=AeroCoeff.C_Y.rud  Table=AeroCoeff.C_Y.Data_rud  InternalRulePriority=Speed  RndMeth=Simplest  InputSameDT=on
  Product{,1..3} (4 alike) : Product
  Sum : Sum  Inputs=+++
  C_y_total : Outport
  wires:
  Sum/1 -> C_y_total/1  "C_y_total"
  Product1/1 -> Sum/1
  Product/1 -> Product1/2  "dYdR"
  Divide/1 -> Product2/1, Product/1
  Bus Selector/1 -> Divide/2  "<WingSpan_m>"
  Gain/1 -> Divide/1
  Bus Selector2/3 -> Gain/1  "<v_m/s>"
  Aircraft_Constant_BUS/1 -> Bus Selector/1
  States_BUS/1 -> Bus Selector2/1
  Product2/1 -> Product3/2  "dYdP"
  Bus Selector2/2 -> Product1/1  "<r_rad/s>"
  Bus Selector2/1 -> Product3/1  "<p_rad/s>"
  Product3/1 -> Sum/2
  Bus Selector3/2 -> LookUp_C_Y_beta/1  "<beta>"
  LookUp_C_Y_rud/1 -> Add1/3
  LookUp_C_Y_ail/1 -> Add1/2
  LookUp_C_Y_beta/1 -> Add1/1
  C_Y0/1 -> Add1/4
  Bus Selector4/1 -> LookUp_C_Y_ail/1  "<Aileron_act>"
  Add1/1 -> Sum/3  "C_Y"
  alpha_beta/1 -> Bus Selector3/1
  prep_Controls_BUS/1 -> Bus Selector4/1
  Bus Selector4/2 -> LookUp_C_Y_rud/1  "<Rudder_act>"
  LookUp_CYp/1 -> Product2/2  "C_Yp"
  Bus Selector3/1 -> LookUp_CYp/1, LookUp_CYr/1  "<alpha>"
  LookUp_CYr/1 -> Product/2  "C_Yr"

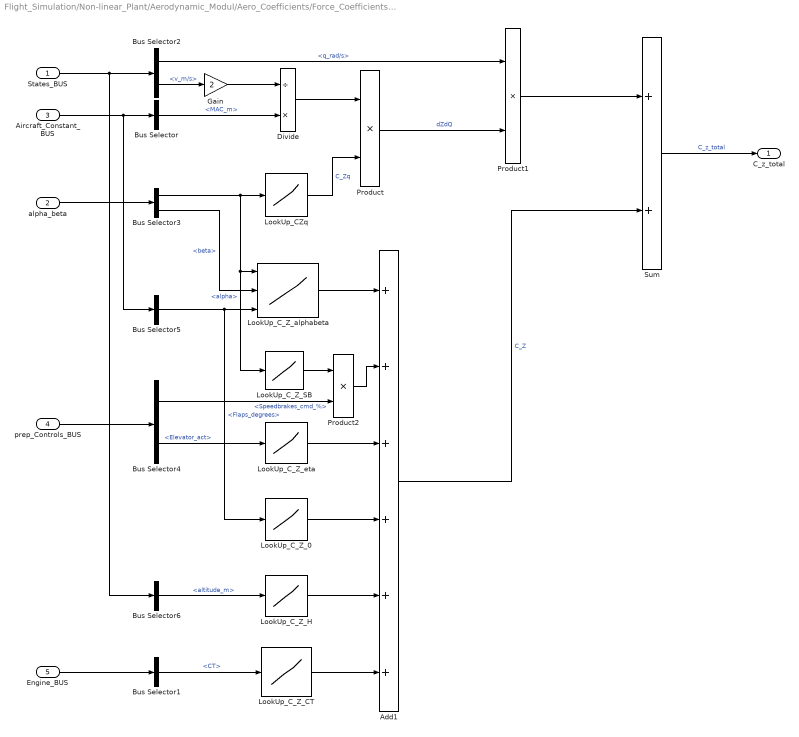
== system Flight_Simulation/Non-linear_Plant/Aerodynamic_Modul/Aero_Coefficients/Force_Coefficients/C_z_total ==
  States_BUS : Inport
  alpha_beta : Inport  Port=2
  Aircraft_Constant_BUS : Inport  Port=3
  prep_Controls_BUS : Inport  Port=4
  Engine_BUS : Inport  Port=5
  Add1 : Sum  Inputs=++++++
  Bus Selector : BusSelector  OutputSignals=Wing_Dimension_BUS.MAC_m
  Bus Selector1 : BusSelector  OutputSignals=CT
  Bus Selector2 : BusSelector  OutputSignals=Rates_p_q_r.q_rad/s,Vel_aero_V_alpha_beta.v_m/s
  Bus Selector3 : BusSelector  OutputSignals=alpha,beta
  Bus Selector4 : BusSelector  OutputSignals=Speedbrakes_cmd_%,Elevator_act
  Bus Selector5 : BusSelector  OutputSignals=Flaps_degrees
  Bus Selector6 : BusSelector  OutputSignals=Position_north_east_alt.altitude_m
  Divide : Product  Inputs=/*
  Gain : Gain  Gain=2
  LookUp_CZq : Lookup_n-D  NumberOfTableDimensions=1  BreakpointsForDimension1=AeroCoeff.C_zq.alpha  Table=AeroCoeff.C_zq.Data  InternalRulePriority=Speed  RndMeth=Simplest  InputSameDT=on
  LookUp_C_Z_0 : Lookup_n-D  NumberOfTableDimensions=1  BreakpointsForDimension1=AeroCoeff.C_Z.Flaps  Table=AeroCoeff.C_Z.Data_0  InternalRulePriority=Speed  RndMeth=Simplest  InputSameDT=on
  LookUp_C_Z_CT : Lookup_n-D  NumberOfTableDimensions=1  BreakpointsForDimension1=AeroCoeff.C_Z_CT  Table=AeroCoeff.C_Z.Data_CT  InternalRulePriority=Speed  RndMeth=Simplest  InputSameDT=on
  LookUp_C_Z_H : Lookup_n-D  NumberOfTableDimensions=1  BreakpointsForDimension1=AeroCoeff.C_Z.h  Table=AeroCoeff.C_Z.Data_H  InternalRulePriority=Speed  RndMeth=Simplest  InputSameDT=on
  LookUp_C_Z_SB : Lookup_n-D  NumberOfTableDimensions=1  BreakpointsForDimension1=AeroCoeff.C_Z.alpha  Table=AeroCoeff.C_Z.Data_sb_alpha  InternalRulePriority=Speed  RndMeth=Simplest  InputSameDT=on
  LookUp_C_Z_alphabeta : Lookup_n-D  NumberOfTableDimensions=3  BreakpointsForDimension1=AeroCoeff.C_Z.alpha  BreakpointsForDimension2=AeroCoeff.C_Z.beta  BreakpointsForDimension3=AeroCoeff.C_Z.Flaps  Table=AeroCoeff.C_Z.Data_alphabeta  InternalRulePriority=Speed  RndMeth=Simplest  InputSameDT=on
      settings: InputPortMap=u0,u1,u2
  LookUp_C_Z_eta : Lookup_n-D  NumberOfTableDimensions=1  BreakpointsForDimension1=AeroCoeff.C_Z.eta  Table=AeroCoeff.C_Z.Data_eta  InternalRulePriority=Speed  RndMeth=Simplest  InputSameDT=on
  Product : Product
  Product1 : Product
  Product2 : Product
  Sum : Sum
  C_z_total : Outport
  wires:
  States_BUS/1 -> Bus Selector6/1, Bus Selector2/1
  Aircraft_Constant_BUS/1 -> Bus Selector5/1, Bus Selector/1
  Bus Selector2/2 -> Gain/1  "<v_m/s>"
  Gain/1 -> Divide/1
  Bus Selector/1 -> Divide/2  "<MAC_m>"
  Divide/1 -> Product/1
  Product/1 -> Product1/2  "dZdQ"
  Add1/1 -> Sum/2  "C_Z"
  Bus Selector2/1 -> Product1/1  "<q_rad/s>"
  Product1/1 -> Sum/1
  Sum/1 -> C_z_total/1  "C_z_total"
  Bus Selector3/1 -> LookUp_C_Z_SB/1, LookUp_C_Z_alphabeta/1, LookUp_CZq/1  "<alpha>"
  LookUp_CZq/1 -> Product/2  "C_Zq"
  alpha_beta/1 -> Bus Selector3/1
  LookUp_C_Z_eta/1 -> Add1/3
  LookUp_C_Z_CT/1 -> Add1/6
  Engine_BUS/1 -> Bus Selector1/1
  LookUp_C_Z_0/1 -> Add1/4
  Bus Selector1/1 -> LookUp_C_Z_CT/1  "<CT>"
  prep_Controls_BUS/1 -> Bus Selector4/1
  Bus Selector4/2 -> LookUp_C_Z_eta/1  "<Elevator_act>"
  Bus Selector3/2 -> LookUp_C_Z_alphabeta/2  "<beta>"
  Bus Selector5/1 -> LookUp_C_Z_0/1, LookUp_C_Z_alphabeta/3  "<Flaps_degrees>"
  Bus Selector6/1 -> LookUp_C_Z_H/1  "<altitude_m>"
  LookUp_C_Z_H/1 -> Add1/5
  LookUp_C_Z_alphabeta/1 -> Add1/1
  LookUp_C_Z_SB/1 -> Product2/1
  Bus Selector4/1 -> Product2/2  "<Speedbrakes_cmd_%>"
  Product2/1 -> Add1/2

== system Flight_Simulation/Non-linear_Plant/Aerodynamic_Modul/Aero_Coefficients/Moment_Coefficients/C_l_total ==
  States_BUS : Inport
  alpha_beta : Inport  Port=2
  Aircraft_Constant_BUS : Inport  Port=3
  prep_Controls_BUS : Inport  Port=4
  Add1 : Sum  Inputs=+++
  Bus Selector : BusSelector  OutputSignals=Wing_Dimension_BUS.WingSpan_m
  Bus Selector2 : BusSelector  OutputSignals=Rates_p_q_r.p_rad/s,Rates_p_q_r.r_rad/s,Vel_aero_V_alpha_beta.v_m/s
  Bus Selector4 : BusSelector  OutputSignals=alpha,beta
  Bus Selector5 : BusSelector  OutputSignals=Aileron_act,Rudder_act
  Divide : Product  Inputs=/*
  Gain : Gain  Gain=2
  LookUp_C_L_Ail : Lookup_n-D  NumberOfTableDimensions=1  BreakpointsForDimension1=AeroCoeff.C_L.ail  Table=AeroCoeff.C_L.Data_ail  InternalRulePriority=Speed  RndMeth=Simplest  InputSameDT=on
  LookUp_C_L_Rud : Lookup_n-D  NumberOfTableDimensions=1  BreakpointsForDimension1=AeroCoeff.C_L.rud  Table=AeroCoeff.C_L.Data_rud  InternalRulePriority=Speed  RndMeth=Simplest  InputSameDT=on
  LookUp_C_L_alphabeta : Lookup_n-D  BreakpointsForDimension1=AeroCoeff.C_L.alpha  BreakpointsForDimension2=AeroCoeff.C_L.beta  Table=AeroCoeff.C_L.Data_alphabeta  InternalRulePriority=Speed  RndMeth=Simplest  InputSameDT=on
      settings: InputPortMap=u0,u1
  LookUp_Clp : Lookup_n-D  NumberOfTableDimensions=1  BreakpointsForDimension1=AeroCoeff.C_lp.alpha  Table=AeroCoeff.C_lp.Data  InternalRulePriority=Speed  RndMeth=Simplest  InputSameDT=on
  LookUp_Clr : Lookup_n-D  NumberOfTableDimensions=1  BreakpointsForDimension1=AeroCoeff.C_lr.alpha  Table=AeroCoeff.C_lr.Data  InternalRulePriority=Speed  RndMeth=Simplest  InputSameDT=on
  LookUp_DLDA : Lookup_n-D  BreakpointsForDimension1=AeroCoeff.DLDA.alpha  BreakpointsForDimension2=AeroCoeff.DLDA.beta  Table=AeroCoeff.DLDA.Data  DiagnosticForOutOfRangeInput=Warning  InternalRulePriority=Speed  RndMeth=Simplest  InputSameDT=on
      settings: InputPortMap=u0,u1
  LookUp_DLDR : Lookup_n-D  BreakpointsForDimension1=AeroCoeff.DLDR.alpha  BreakpointsForDimension2=AeroCoeff.DLDR.beta  Table=AeroCoeff.DLDR.Data  DiagnosticForOutOfRangeInput=Warning  InternalRulePriority=Speed  RndMeth=Simplest  InputSameDT=on
      settings: InputPortMap=u0,u1
  Product{,1..2,4..6} (6 alike) : Product
  Sum : Sum  Inputs=+++++
  C_l_total : Outport
  wires:
  States_BUS/1 -> Bus Selector2/1
  Aircraft_Constant_BUS/1 -> Bus Selector/1
  Bus Selector2/3 -> Gain/1  "<v_m/s>"
  Gain/1 -> Divide/1
  Bus Selector/1 -> Divide/2  "<WingSpan_m>"
  Divide/1 -> Product/1, Product2/1
  Product/1 -> Product1/2  "dLdR"
  Product1/1 -> Sum/1
  Sum/1 -> C_l_total/1  "C_l_total"
  Add1/1 -> Sum/5  "C_L"
  Bus Selector2/2 -> Product1/1  "<r_rad/s>"
  Product2/1 -> Product4/2  "dLdP"
  Bus Selector2/1 -> Product4/1  "<p_rad/s>"
  Product4/1 -> Sum/2
  LookUp_DLDA/1 -> Product5/2  "DLDA"
  Product5/1 -> Sum/3
  Bus Selector5/2 -> LookUp_C_L_Rud/1, Product6/1  "<Rudder_act>"
  LookUp_DLDR/1 -> Product6/2  "DLDR"
  Product6/1 -> Sum/4
  alpha_beta/1 -> Bus Selector4/1
  prep_Controls_BUS/1 -> Bus Selector5/1
  Bus Selector5/1 -> LookUp_C_L_Ail/1, Product5/1  "<Aileron_act>"
  LookUp_Clp/1 -> Product2/2  "C_lp"
  LookUp_Clr/1 -> Product/2  "C_lr"
  Bus Selector4/1 -> LookUp_C_L_alphabeta/1, LookUp_DLDR/1, LookUp_DLDA/1, LookUp_Clp/1, LookUp_Clr/1  "<alpha>"
  Bus Selector4/2 -> LookUp_C_L_alphabeta/2, LookUp_DLDR/2, LookUp_DLDA/2  "<beta>"
  LookUp_C_L_alphabeta/1 -> Add1/1  "C_L"
  LookUp_C_L_Rud/1 -> Add1/3
  LookUp_C_L_Ail/1 -> Add1/2

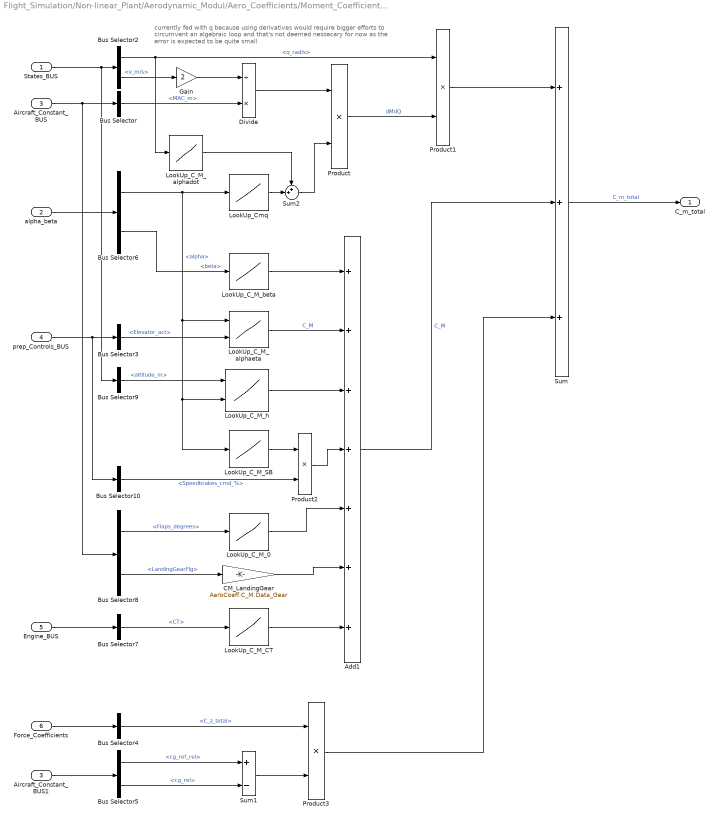
== system Flight_Simulation/Non-linear_Plant/Aerodynamic_Modul/Aero_Coefficients/Moment_Coefficients/C_m_total ==
  note: currently fed with q because using derivatives would require bigger efforts
      | to circumvent an algebraic loop and that's not deemed nessecary for now
      | as the error is expected to be quite small
  States_BUS : Inport
  alpha_beta : Inport  Port=2
  Aircraft_Constant_BUS : Inport  Port=3
  prep_Controls_BUS : Inport  Port=4
  Engine_BUS : Inport  Port=5
  Force_Coefficients : Inport  Port=6
  Add1 : Sum  Inputs=+++++++
  Aircraft_Constant_BUS1 : InportShadow  Port=3
  Bus Selector : BusSelector  OutputSignals=Wing_Dimension_BUS.MAC_m
  Bus Selector10 : BusSelector  OutputSignals=Speedbrakes_cmd_%
  Bus Selector2 : BusSelector  OutputSignals=Rates_p_q_r.q_rad/s,Vel_aero_V_alpha_beta.v_m/s
  Bus Selector3 : BusSelector  OutputSignals=Elevator_act
  Bus Selector4 : BusSelector  OutputSignals=C_z_total
  Bus Selector5 : BusSelector  OutputSignals=cg_BUS.cg_ref_rel,cg_BUS.cg_rel
  Bus Selector6 : BusSelector  OutputSignals=alpha,beta
  Bus Selector7 : BusSelector  OutputSignals=CT
  Bus Selector8 : BusSelector  OutputSignals=Flaps_degrees,LandingGearFlg
  Bus Selector9 : BusSelector  OutputSignals=Position_north_east_alt.altitude_m
  CM_LandingGear : Gain  Gain=AeroCoeff.C_M.Data_Gear
  Divide : Product  Inputs=/*
  Gain : Gain  Gain=2
  LookUp_C_M_0 : Lookup_n-D  NumberOfTableDimensions=1  BreakpointsForDimension1=AeroCoeff.C_M.Flaps  Table=AeroCoeff.C_M.Data_0  InternalRulePriority=Speed  RndMeth=Simplest  InputSameDT=on
  LookUp_C_M_CT : Lookup_n-D  NumberOfTableDimensions=1  BreakpointsForDimension1=AeroCoeff.C_M.CT  Table=AeroCoeff.C_M.Data_CT  InternalRulePriority=Speed  RndMeth=Simplest  InputSameDT=on
  LookUp_C_M_SB : Lookup_n-D  NumberOfTableDimensions=1  BreakpointsForDimension1=AeroCoeff.C_M.alpha  Table=AeroCoeff.C_M.Data_sb_alpha  InternalRulePriority=Speed  RndMeth=Simplest  InputSameDT=on
  LookUp_C_M_alphadot : Lookup_n-D  NumberOfTableDimensions=1  BreakpointsForDimension1=AeroCoeff.C_M.alphadot  Table=AeroCoeff.C_M.Data_alphadot  InternalRulePriority=Speed  RndMeth=Simplest  InputSameDT=on
  LookUp_C_M_alphaeta : Lookup_n-D  BreakpointsForDimension1=AeroCoeff.C_M.alpha  BreakpointsForDimension2=AeroCoeff.C_M.eta  Table=AeroCoeff.C_M.Data_alphaeta  InternalRulePriority=Speed  RndMeth=Simplest  InputSameDT=on
      settings: InputPortMap=u0,u1
  LookUp_C_M_beta : Lookup_n-D  NumberOfTableDimensions=1  BreakpointsForDimension1=AeroCoeff.C_M.beta  Table=AeroCoeff.C_M.Data_beta  InternalRulePriority=Speed  RndMeth=Simplest  InputSameDT=on
  LookUp_C_M_h : Lookup_n-D  BreakpointsForDimension1=AeroCoeff.C_M.h  BreakpointsForDimension2=AeroCoeff.C_M.h_alpha  Table=AeroCoeff.C_M.Data_H_alpha  InternalRulePriority=Speed  RndMeth=Simplest  InputSameDT=on
      settings: InputPortMap=u0,u1
  LookUp_Cmq : Lookup_n-D  NumberOfTableDimensions=1  BreakpointsForDimension1=AeroCoeff.C_mq.alpha  Table=AeroCoeff.C_mq.Data  InternalRulePriority=Speed  RndMeth=Simplest  InputSameDT=on
  Product{,1..3} (4 alike) : Product
  Sum : Sum  Inputs=+++
  Sum1 : Sum  Inputs=+-
  Sum2 : Sum  Inputs=++|
  C_m_total : Outport
  wires:
  States_BUS/1 -> Bus Selector2/1, Bus Selector9/1
  Aircraft_Constant_BUS/1 -> Bus Selector8/1, Bus Selector/1
  LookUp_Cmq/1 -> Sum2/2
  Bus Selector2/2 -> Gain/1  "<v_m/s>"
  Gain/1 -> Divide/1
  Bus Selector/1 -> Divide/2  "<MAC_m>"
  Divide/1 -> Product/1
  Product/1 -> Product1/2  "dMdQ"
  Add1/1 -> Sum/2  "C_M"
  Bus Selector2/1 -> Product1/1, LookUp_C_M_alphadot/1  "<q_rad/s>"
  Sum/1 -> C_m_total/1  "C_m_total"
  Force_Coefficients/1 -> Bus Selector4/1
  Bus Selector4/1 -> Product3/1  "<C_z_total>"
  Aircraft_Constant_BUS1/1 -> Bus Selector5/1
  Sum1/1 -> Product3/2
  Bus Selector3/1 -> LookUp_C_M_alphaeta/2  "<Elevator_act>"
  Product1/1 -> Sum/1
  Product3/1 -> Sum/3
  prep_Controls_BUS/1 -> Bus Selector10/1, Bus Selector3/1
  Engine_BUS/1 -> Bus Selector7/1
  alpha_beta/1 -> Bus Selector6/1
  Bus Selector6/1 -> LookUp_C_M_h/2, LookUp_C_M_SB/1, LookUp_C_M_alphaeta/1, LookUp_Cmq/1  "<alpha>"
  Bus Selector7/1 -> LookUp_C_M_CT/1  "<CT>"
  LookUp_C_M_alphaeta/1 -> Add1/2  "C_M"
  LookUp_C_M_CT/1 -> Add1/7
  LookUp_C_M_beta/1 -> Add1/1
  Bus Selector6/2 -> LookUp_C_M_beta/1  "<beta>"
  LookUp_C_M_0/1 -> Add1/5
  CM_LandingGear/1 -> Add1/6
  LookUp_C_M_alphadot/1 -> Sum2/1
  Sum2/1 -> Product/2
  Bus Selector8/1 -> LookUp_C_M_0/1  "<Flaps_degrees>"
  Bus Selector9/1 -> LookUp_C_M_h/1  "<altitude_m>"
  Bus Selector5/1 -> Sum1/1  "<cg_ref_rel>"
  Bus Selector5/2 -> Sum1/2  "<cg_rel>"
  Bus Selector10/1 -> Product2/2  "<Speedbrakes_cmd_%>"
  LookUp_C_M_SB/1 -> Product2/1
  Bus Selector8/2 -> CM_LandingGear/1  "<LandingGearFlg>"
  Product2/1 -> Add1/4
  LookUp_C_M_h/1 -> Add1/3

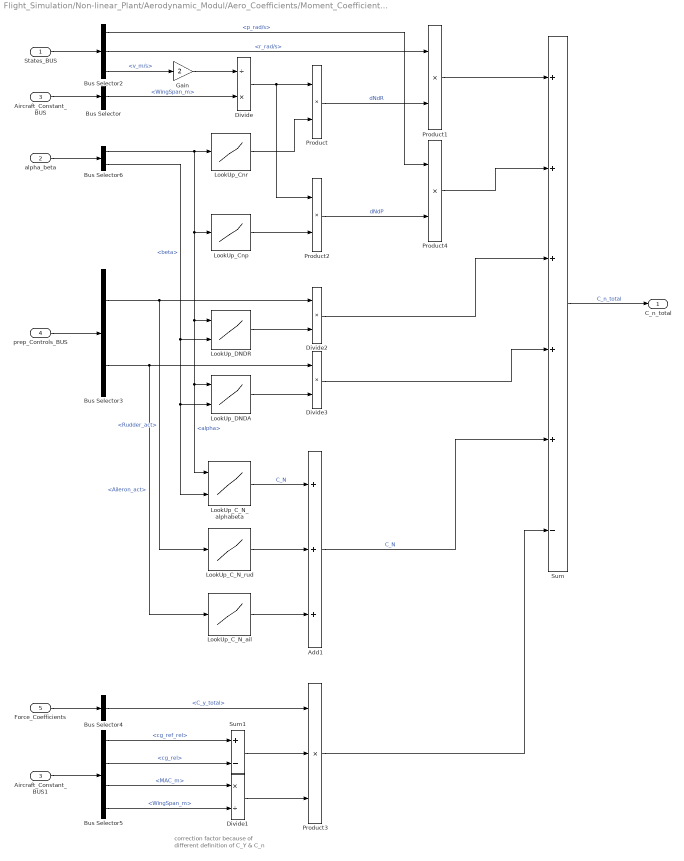
== system Flight_Simulation/Non-linear_Plant/Aerodynamic_Modul/Aero_Coefficients/Moment_Coefficients/C_n_total ==
  note: correction factor because of
      | different definition of C_Y & C_n
  States_BUS : Inport
  alpha_beta : Inport  Port=2
  Aircraft_Constant_BUS : Inport  Port=3
  prep_Controls_BUS : Inport  Port=4
  Force_Coefficients : Inport  Port=5
  Add1 : Sum  Inputs=+++
  Aircraft_Constant_BUS1 : InportShadow  Port=3
  Bus Selector : BusSelector  OutputSignals=Wing_Dimension_BUS.WingSpan_m
  Bus Selector2 : BusSelector  OutputSignals=Rates_p_q_r.p_rad/s,Rates_p_q_r.r_rad/s,Vel_aero_V_alpha_beta.v_m/s
  Bus Selector3 : BusSelector  OutputSignals=Rudder_act,Aileron_act
  Bus Selector4 : BusSelector  OutputSignals=C_y_total
  Bus Selector5 : BusSelector  OutputSignals=cg_BUS.cg_ref_rel,cg_BUS.cg_rel,Wing_Dimension_BUS.MAC_m,Wing_Dimension_BUS.WingSpan_m
  Bus Selector6 : BusSelector  OutputSignals=alpha,beta
  Divide : Product  Inputs=/*
  Divide1 : Product  Inputs=*/
  Divide2 : Product
  Divide3 : Product
  Gain : Gain  Gain=2
  LookUp_C_N_ail : Lookup_n-D  NumberOfTableDimensions=1  BreakpointsForDimension1=AeroCoeff.C_N.ail  Table=AeroCoeff.C_N.Data_ail  InternalRulePriority=Speed  RndMeth=Simplest  InputSameDT=on
  LookUp_C_N_alphabeta : Lookup_n-D  BreakpointsForDimension1=AeroCoeff.C_N.alpha  BreakpointsForDimension2=AeroCoeff.C_N.beta  Table=AeroCoeff.C_N.Data_alphabeta  InternalRulePriority=Speed  RndMeth=Simplest  InputSameDT=on
      settings: InputPortMap=u0,u1
  LookUp_C_N_rud : Lookup_n-D  NumberOfTableDimensions=1  BreakpointsForDimension1=AeroCoeff.C_N.rud  Table=AeroCoeff.C_N.Data_rud  InternalRulePriority=Speed  RndMeth=Simplest  InputSameDT=on
  LookUp_Cnp : Lookup_n-D  NumberOfTableDimensions=1  BreakpointsForDimension1=AeroCoeff.C_np.alpha  Table=AeroCoeff.C_np.Data  InternalRulePriority=Speed  RndMeth=Simplest  InputSameDT=on
  LookUp_Cnr : Lookup_n-D  NumberOfTableDimensions=1  BreakpointsForDimension1=AeroCoeff.C_nr.alpha  Table=AeroCoeff.C_nr.Data  InternalRulePriority=Speed  RndMeth=Simplest  InputSameDT=on
  LookUp_DNDA : Lookup_n-D  BreakpointsForDimension1=AeroCoeff.DNDA.alpha  BreakpointsForDimension2=AeroCoeff.DNDA.beta  Table=AeroCoeff.DNDA.Data  DiagnosticForOutOfRangeInput=Warning  InternalRulePriority=Speed  RndMeth=Simplest  InputSameDT=on
      settings: InputPortMap=u0,u1
  LookUp_DNDR : Lookup_n-D  BreakpointsForDimension1=AeroCoeff.DNDR.alpha  BreakpointsForDimension2=AeroCoeff.DNDR.beta  Table=AeroCoeff.DNDR.Data  DiagnosticForOutOfRangeInput=Warning  InternalRulePriority=Speed  RndMeth=Simplest  InputSameDT=on
      settings: InputPortMap=u0,u1
  Product{,1..2,4} (4 alike) : Product
  Product3 : Product  Inputs=3
  Sum : Sum  Inputs=+++++-
  Sum1 : Sum  Inputs=+-
  C_n_total : Outport
  wires:
  States_BUS/1 -> Bus Selector2/1
  Aircraft_Constant_BUS/1 -> Bus Selector/1
  LookUp_Cnr/1 -> Product/2
  Bus Selector2/3 -> Gain/1  "<v_m/s>"
  Gain/1 -> Divide/1
  Bus Selector/1 -> Divide/2  "<WingSpan_m>"
  Divide/1 -> Product/1, Product2/1
  Product/1 -> Product1/2  "dNdR"
  LookUp_Cnp/1 -> Product2/2
  Product1/1 -> Sum/1
  Sum/1 -> C_n_total/1  "C_n_total"
  Force_Coefficients/1 -> Bus Selector4/1
  Bus Selector4/1 -> Product3/1  "<C_y_total>"
  Aircraft_Constant_BUS1/1 -> Bus Selector5/1
  Bus Selector5/1 -> Sum1/1  "<cg_ref_rel>"
  Bus Selector5/2 -> Sum1/2  "<cg_rel>"
  Sum1/1 -> Product3/2
  Product2/1 -> Product4/2  "dNdP"
  Bus Selector2/2 -> Product1/1  "<r_rad/s>"
  Bus Selector2/1 -> Product4/1  "<p_rad/s>"
  Product4/1 -> Sum/2
  Add1/1 -> Sum/5  "C_N"
  Bus Selector5/3 -> Divide1/1  "<MAC_m>"
  Bus Selector5/4 -> Divide1/2  "<WingSpan_m>"
  Divide1/1 -> Product3/3
  LookUp_DNDR/1 -> Divide2/2
  Bus Selector3/1 -> LookUp_C_N_rud/1, Divide2/1  "<Rudder_act>"
  Divide2/1 -> Sum/3
  LookUp_DNDA/1 -> Divide3/2
  Bus Selector3/2 -> LookUp_C_N_ail/1, Divide3/1  "<Aileron_act>"
  Divide3/1 -> Sum/4
  Product3/1 -> Sum/6
  prep_Controls_BUS/1 -> Bus Selector3/1
  alpha_beta/1 -> Bus Selector6/1
  Bus Selector6/1 -> LookUp_C_N_alphabeta/1, LookUp_DNDA/1, LookUp_DNDR/1, LookUp_Cnp/1, LookUp_Cnr/1  "<alpha>"
  Bus Selector6/2 -> LookUp_C_N_alphabeta/2, LookUp_DNDA/2, LookUp_DNDR/2  "<beta>"
  LookUp_C_N_rud/1 -> Add1/2
  LookUp_C_N_alphabeta/1 -> Add1/1  "C_N"
  LookUp_C_N_ail/1 -> Add1/3

== matlab function Flight_Simulation/Environment_Subsystems/ISA_StandardAtmosphere_Model_ScriptVersion/ISA_Standard_Atmosphere_Model ==
  data: p_static output; q_bar output; rho output; T output; Mach output; H input; V input; g input; R input; compressibility input
function [p_static,q_bar,rho,T,Mach]  = ISA_StandardAtmosphere(H,V,g,R,compressibility)


% --- Units ---
% H - m
% T - °K
% p - Pa
% rho - kg/m^3
% R - J/(kg*K)

k = 1.4;

% Set constants needed for cascadic atmosphere calculation
if H <= 11000
    
    H_A     = 0;
    beta    = -0.0065;
    T_A     = 288.15;
    p_A     = 101325;
    rho_A   = 1.225;
    
elseif H > 11000 && H <= 20000
    
    H_A     = 11000;
    beta    = 1; %to avoid division by zero, will not be used anyway
    T_A     = 216.65;
    p_A     = 22620;
    rho_A   = 0.3637;
    
else
    
    H_A     = 20000;
    beta    = 0.001;
    T_A     = 216.65;
    p_A     = 5469;
    rho_A   = 0.0879;

end       

%% Equations
if H > 11000 && H <= 20000
    
    T = T_A;
    p_static = p_A * exp(-(g/R)*((H - H_A)/T_A));
    rho = rho_A * exp(-(g/R)*((H - H_A)/T_A));

else
    
    T = T_A + beta*(H - H_A);
    p_static = p_A * (1 + (beta/T_A) * (H - H_A))^(-g/(R*beta));
    rho = rho_A * (1 + (beta/T_A) * (H - H_A))^(-(g/(R*beta))-1);
    
end

% rho = 1.2257; % only for ONERA validation
% T = 288.15+15; % only for ONERA validation

a = sqrt(k*R*T);
Mach = V/a;

if compressibility == 1
    % compressible flow
    q_bar = p_static*( (1+ (k-1)/2 *Mach^2 )^( k/(k-1) ) -1 );
else
    % incompressible flow
    q_bar = 0.5 .* rho .* V.^2;
end

end
